simulink model "part1_3"  (R2023b)
settings: Solver=VariableStepAuto  StartTime=0.0  StopTime=10.0  RelTol=1e-3
settings Model: Creator=Zahedi  LastModifiedBy=Zahedi

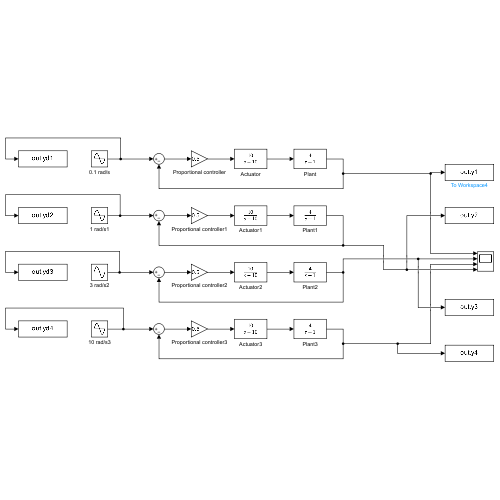
[thumbnail: Simulink's stored preview of the top-level diagram]
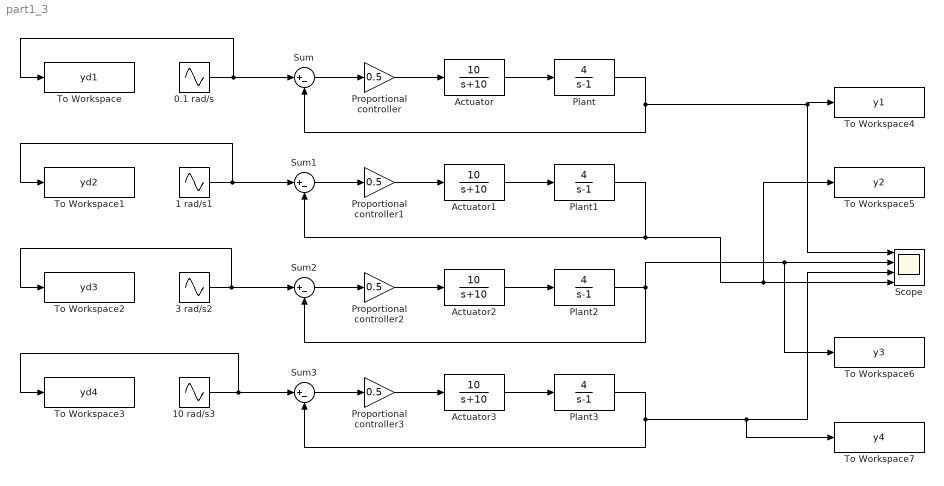
== system part1_3 ==
  0.1 rad/s : Sin  Frequency=0.1  SampleTime=0
  1 rad/s1 : Sin  SampleTime=0
  10 rad/s3 : Sin  Frequency=10  SampleTime=0
  3 rad/s2 : Sin  Frequency=3  SampleTime=0
  Actuator{,1..3} (4 alike) : TransferFcn  Numerator=[10]  Denominator=[1 10]
  Plant{,1..3} (4 alike) : TransferFcn  Numerator=[4]  Denominator=[1 -1]
  Proportional controller{,1..3} (4 alike) : Gain  Gain=0.5
  Scope : Scope  NumInputPorts=4
  Sum{,1..3} (4 alike) : Sum  Inputs=|+-
  To Workspace : ToWorkspace  VariableName=yd1  SaveFormat=Timeseries  SampleTime=-1
  To Workspace1 : ToWorkspace  VariableName=yd2  SaveFormat=Timeseries  SampleTime=-1
  To Workspace2 : ToWorkspace  VariableName=yd3  SaveFormat=Timeseries  SampleTime=-1
  To Workspace3 : ToWorkspace  VariableName=yd4  SaveFormat=Timeseries  SampleTime=-1
  To Workspace4 : ToWorkspace  VariableName=y1  SaveFormat=Timeseries  SampleTime=-1
  To Workspace5 : ToWorkspace  VariableName=y2  SaveFormat=Timeseries  SampleTime=-1
  To Workspace6 : ToWorkspace  VariableName=y3  SaveFormat=Timeseries  SampleTime=-1
  To Workspace7 : ToWorkspace  VariableName=y4  SaveFormat=Timeseries  SampleTime=-1
  wires:
  Actuator/1 -> Plant/1
  Proportional controller/1 -> Actuator/1
  Plant/1 -> To Workspace4/1, Scope/1, Sum/2
  Sum/1 -> Proportional controller/1
  0.1 rad/s/1 -> To Workspace/1, Sum/1
  Actuator1/1 -> Plant1/1
  Sum1/1 -> Proportional controller1/1
  Proportional controller1/1 -> Actuator1/1
  Plant1/1 -> To Workspace5/1, Scope/4, Sum1/2
  1 rad/s1/1 -> To Workspace1/1, Sum1/1
  Actuator2/1 -> Plant2/1
  Sum2/1 -> Proportional controller2/1
  Proportional controller2/1 -> Actuator2/1
  Plant2/1 -> To Workspace6/1, Scope/2, Sum2/2
  3 rad/s2/1 -> To Workspace2/1, Sum2/1
  Actuator3/1 -> Plant3/1
  Sum3/1 -> Proportional controller3/1
  Proportional controller3/1 -> Actuator3/1
  Plant3/1 -> To Workspace7/1, Scope/3, Sum3/2
  10 rad/s3/1 -> To Workspace3/1, Sum3/1
